simulink model "sim_esttimated_speed_model"  (R2017b)
settings: Solver=VariableStepAuto  StartTime=0.0  StopTime=tstop  RelTol=1e-3
values from neighbouring files (symbols this model uses):
  tsamp = 100    [analyse_dynamics_v3.m]    (also in run_task_1_8.m = 10; system_identification.m)
undefined symbols (not defined in the file or in its folder): K_v, n_c, T1, T2
settings Model: Creator=Alexandra  LastModifiedBy=Alexandra

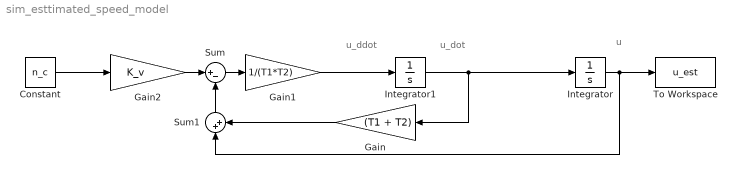
== system sim_esttimated_speed_model ==
  note: u
  note: u_ddot
  note: u_dot
  Constant : Constant  Value=n_c
  Gain : Gain  Gain=(T1 + T2)
  Gain1 : Gain  Gain=1/(T1*T2)
  Gain2 : Gain  Gain=K_v
  Integrator : Integrator  InitialCondition=6.63
  Integrator1 : Integrator
  Sum : Sum  Inputs=|+-
  Sum1 : Sum  Inputs=|++
  To Workspace : ToWorkspace  VariableName=u_est  SaveFormat=Structure With Time  SampleTime=tsamp
  wires:
  Constant/1 -> Gain2/1
  Gain2/1 -> Sum/1
  Sum/1 -> Gain1/1
  Gain1/1 -> Integrator1/1
  Sum1/1 -> Sum/2
  Gain/1 -> Sum1/2
  Integrator1/1 -> Gain/1, Integrator/1
  Integrator/1 -> To Workspace/1, Sum1/1
